simulink model "launcher_simulation"  (R2025b)
settings: Solver=VariableStepAuto  StartTime=0.0  StopTime=5  RelTol=1e-3
values from neighbouring files (symbols this model uses):
  C_d = 0.4    [initial_params.m]
  C_l = 0.2    [initial_params.m]
  C_m = 0.01    [initial_params.m]
  g = 9.81    [initial_params.m]
  k_lift = 1.2    [initial_params.m]
  rho = 1.225    [initial_params.m]
undefined symbols (not defined in the file or in its folder): Initial_Height, mass, omega_0, radius, V_0
settings Model: SimulationMode=rapid-accelerator  Creator=Eilon  LastModifiedBy=Eilon

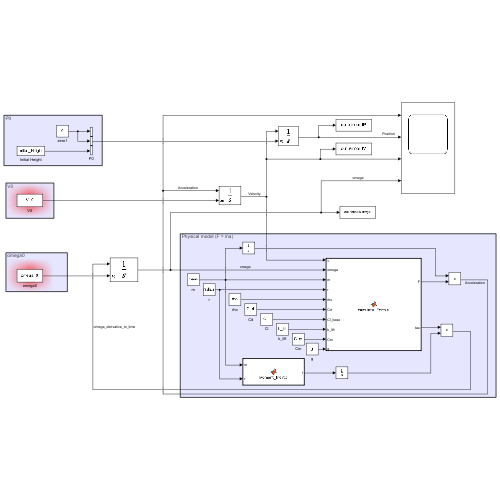
[thumbnail: Simulink's stored preview of the top-level diagram]
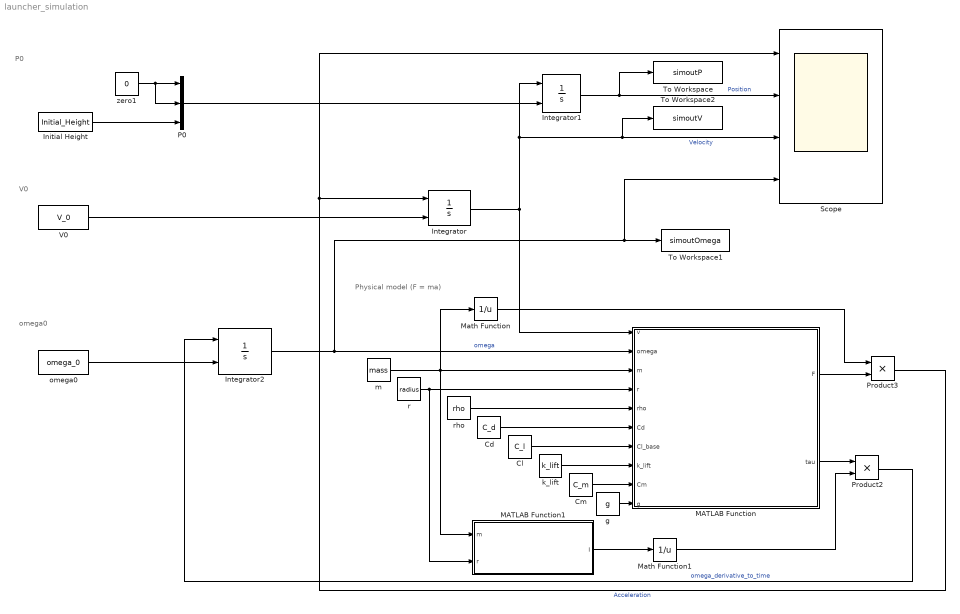
== system launcher_simulation ==
  note: Physical model (F = ma)
  note: V0
  note: P0
  note: omega0
  Cd : Constant  Value=C_d
  Cl : Constant  Value=C_l
  Cm : Constant  Value=C_m
  Initial Height : Constant  Value=Initial_Height
  Integrator : Integrator  InitialConditionSource=external
  Integrator1 : Integrator  InitialConditionSource=external
  Integrator2 : Integrator  InitialConditionSource=external
  MATLAB Function : MATLAB Function  TreatAsAtomicUnit=on
  MATLAB Function1 : MATLAB Function  TreatAsAtomicUnit=on
  Math Function : Math  Operator=reciprocal
  Math Function1 : Math  Operator=reciprocal
  P0 : Concatenate  NumInputs=3
  Product2 : Product
  Product3 : Product
  Scope : Scope  NumInputPorts=4
      settings: ActiveDisplayYMinimum=-81.3942383913958  ActiveDisplayYMaximum=122.50735054986983
  To Workspace : ToWorkspace  VariableName=simoutP  SaveFormat=Timeseries  SampleTime=-1
  To Workspace1 : ToWorkspace  VariableName=simoutOmega  SaveFormat=Timeseries  SampleTime=-1
  To Workspace2 : ToWorkspace  VariableName=simoutV  SaveFormat=Timeseries  SampleTime=-1
  V0 : Constant  Value=V_0
  g : Constant  Value=g
  k_lift : Constant  Value=k_lift
  m : Constant  Value=mass
  omega0 : Constant  Value=omega_0
  r : Constant  Value=radius
  rho : Constant  Value=rho
  zero1 : Constant  Value=0
  wires:
  Integrator/1 -> Integrator1/1, To Workspace2/1, Scope/3, MATLAB Function/1(v)  "Velocity"
  Product3/1 -> Scope/1, Integrator/1  "Acceleration"
  Integrator1/1 -> To Workspace/1, Scope/2  "Position"
  g/1 -> MATLAB Function/10(g)
  r/1 -> MATLAB Function1/2(r), MATLAB Function/4(r)
  m/1 -> MATLAB Function1/1(m), MATLAB Function/3(m), Math Function/1
  omega0/1 -> Integrator2/2
  Cd/1 -> MATLAB Function/6(Cd)
  Cl/1 -> MATLAB Function/7(Cl_base)
  rho/1 -> MATLAB Function/5(rho)
  zero1/1 -> P0/2, P0/1
  P0/1 -> Integrator1/2
  Initial Height/1 -> P0/3
  Integrator2/1 -> MATLAB Function/2(omega), Scope/4, To Workspace1/1  "omega"
  Math Function/1 -> Product3/1
  MATLAB Function/1(F) -> Product3/2
  Cm/1 -> MATLAB Function/9(Cm)
  Product2/1 -> Integrator2/1  "omega_derivative_to_time"
  MATLAB Function1/1(I) -> Math Function1/1
  MATLAB Function/2(tau) -> Product2/1
  Math Function1/1 -> Product2/2
  k_lift/1 -> MATLAB Function/8(k_lift)
  V0/1 -> Integrator/2

== matlab function launcher_simulation/MATLAB Function1 ==
  data: I output; m input; r input
function I = Moment_Inertia(m, r)
    % חישוב מומנט אינרציה (עבור כדור מלא)
    I = (2/5) * m * r^2;
end

== matlab function launcher_simulation/MATLAB Function ==
  data: v input; F output; omega input; m input; r input; rho input; Cd input; Cl_base input; k_lift input; Cm input; g input; tau output
function [F, tau] = calculate_Forces(v, omega, m, r, rho, Cd, Cl_base, k_lift, Cm, g)
    v = v(:); 
    omega = omega(:);
    v_mag = norm(v);
    
    A = pi * r^2;
    
    % הגנה מפני חילוק באפס
    if v_mag > 1e-3
        S = (norm(omega) * r) / v_mag;
        % מודל לא-ליניארי משופר (Power Law)
        % Cl_base כאן מייצג את המקדם המקסימלי האפשרי
        Cl_dynamic = Cl_base * (1 - exp(-k_lift * S)); 
    else
        Cl_dynamic = 0;
    end
    
    % חישוב כוחות
    Fg = [0; 0; -m*g];
    Fd = -0.5 * rho * Cd * A * v_mag * v; % וקטור גרר
    
    % שימוש בוקטור יחידה לכיוון כוח מגנוס
    omega_cross_v = cross(omega, v);
    if norm(omega_cross_v) > 1e-6
        Fm_dir = omega_cross_v / norm(omega_cross_v);
        Fm = 0.5 * rho * (v_mag^2) * Cl_dynamic * A * Fm_dir;
    else
        Fm = [0;0;0];
    end
    
    F = Fg + Fd + Fm;
    tau = -0.5 * rho * v_mag * Cm * (r^4) * omega;
end
